simulink model "HW2_FSR_ES3_Almost_NonLinear"  (R2023b)
settings: Solver=ode23  StartTime=0.0  StopTime=T  FixedStep=0.001  RelTol=1e-5
values from neighbouring files (symbols this model uses):
  c = 36/r^0.3    (= 36)    [HW2_FSR_ES3.m]
  k_2_a = 3*c^2/r    (= 3888)    [HW2_FSR_ES3.m]
  r = 1    [HW2_FSR_ES3.m]
libraries: robotmobilelib x1
settings Model: Creator=emman  LastModifiedBy=emman

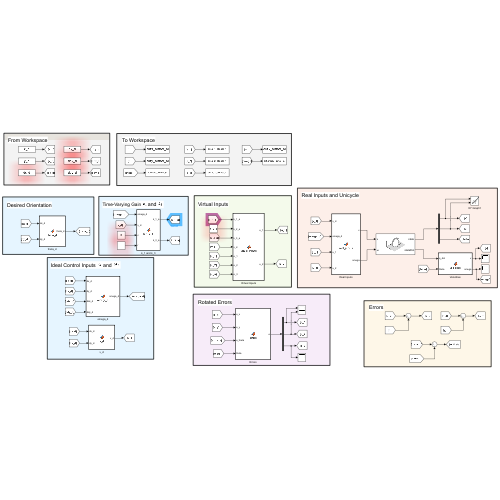
[thumbnail: Simulink's stored preview of the top-level diagram]
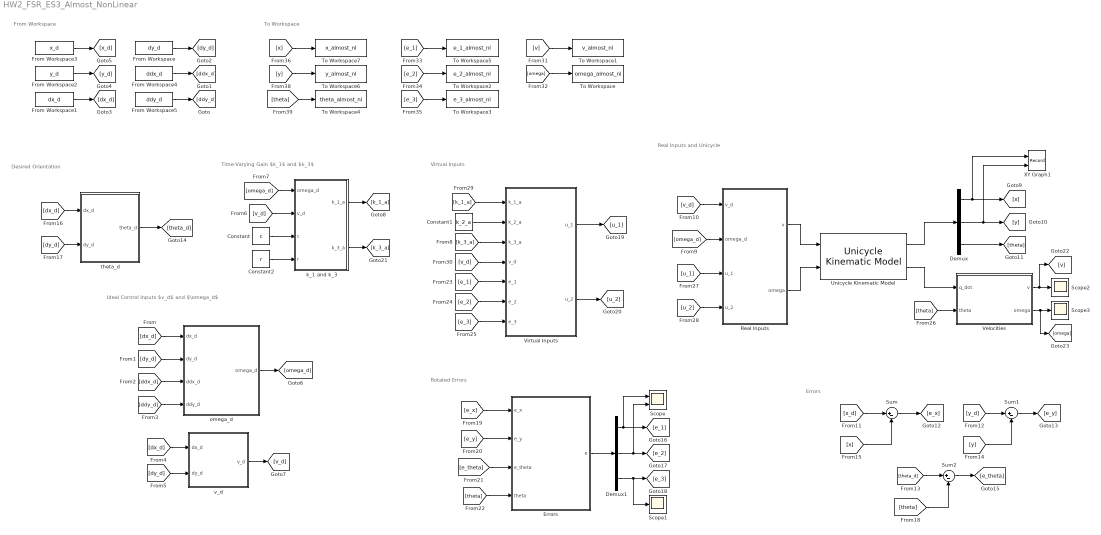
== system HW2_FSR_ES3_Almost_NonLinear ==
  note: To Workspace
  note: From Workspace
  note: Desired Orientation
  note: Rotated Errors
  note: Ideal Control Inputs $v_d$ and $\omega_d$
  note: Time-Varying Gain $k_1$ and $k_3$
  note: Virtual Inputs
  note: Real Inputs and Unicycle
  note: Errors
  Constant : Constant  Value=c
  Constant1 : Constant  Value=k_2_a
  Constant2 : Constant  Value=r
  Demux : Demux  Outputs=3
  Demux1 : Demux  Outputs=3
  Errors : MATLAB Function  TreatAsAtomicUnit=on
  From Workspace : FromWorkspace  VariableName=dy_d
  From Workspace1 : FromWorkspace  VariableName=dx_d
  From Workspace2 : FromWorkspace  VariableName=y_d
  From Workspace3 : FromWorkspace  VariableName=x_d
  From Workspace4 : FromWorkspace  VariableName=ddx_d
  From Workspace5 : FromWorkspace  VariableName=ddy_d
  Real Inputs : MATLAB Function  TreatAsAtomicUnit=on
  Scope : Scope  NumInputPorts=2
  Scope1 : Scope
  Scope2 : Scope
  Scope3 : Scope
  Sum : Sum  Inputs=|+-
  Sum1 : Sum  Inputs=|+-
  Sum2 : Sum  Inputs=|+-
  To Workspace : ToWorkspace  VariableName=omega_almost_nl  SaveFormat=Timeseries  SampleTime=-1
  To Workspace1 : ToWorkspace  VariableName=v_almost_nl  SaveFormat=Timeseries  SampleTime=-1
  To Workspace2 : ToWorkspace  VariableName=e_2_almost_nl  SaveFormat=Timeseries  SampleTime=-1
  To Workspace3 : ToWorkspace  VariableName=e_3_almost_nl  SaveFormat=Timeseries  SampleTime=-1
  To Workspace4 : ToWorkspace  VariableName=theta_almost_nl  SaveFormat=Timeseries  SampleTime=-1
  To Workspace5 : ToWorkspace  VariableName=e_1_almost_nl  SaveFormat=Timeseries  SampleTime=-1
  To Workspace6 : ToWorkspace  VariableName=y_almost_nl  SaveFormat=Timeseries  SampleTime=-1
  To Workspace7 : ToWorkspace  VariableName=x_almost_nl  SaveFormat=Timeseries  SampleTime=-1
  Unicycle Kinematic Model : robotmobilelib/Unicycle Kinematic Model  VehicleInputs=Vehicle Speed & Heading Angular Velocity  WheelRadius=0.1  WheelSpeedRange=[-Inf Inf]  InitialState=q_i  SimulateUsing=Interpreted execution
  Velocities : MATLAB Function  TreatAsAtomicUnit=on
  Virtual Inputs : MATLAB Function  TreatAsAtomicUnit=on
  XY Graph1 : Record  FileSettingsInternal="{\"entries\":[{\"content\":{\"excelSettings\":{\"content\":{},\"type\":\"Streamout.ExcelSettings\"}},\"type\":\"Streamout.FileSettingStorage\",\"uuid\":\"\"}],\"packageUris\":[\"http:\\/\\/schema.mathworks.com\\/mf0\\/streamout_blocks\\/R2020a\"],\"version\":\"1.0\"}"  Layout=[1 1]  SignalsInternal="{\"entries\":[{\"content\":{\"signals\":[{\"content\":{\"blockPath\":[],\"dimensions\":[1],\"domain\":\"\",\"lineColor\":\"#77ac30\",\"plots\":[1],\"port\":1,\"sid\":[\"\"],\"signalID\":6338,\"signalName\":\"Demux:1\"},\"type\":\"RecordBlkView.Signal\",\"uuid\":\"\"},{\"content\":{\"blockPath\":[],\"dimensions\":[1],\"domain\":\"\",\"lineColor\":\"#4dbeee\",\"plots\":[1],\"port\":2,\"sid\":[\"\"],\"signalID\":6342,\"signalName\":\"Demux:2\"},\"type\":\"RecordBlkView.Signal\",\"uuid\":\"\"}]},\"type\":\"RecordBlkView.InputSignals\",\"uuid\":\"\"}],\"packageUris\":[\"http:\\/\\/schema.mathworks.com\\/mf0\\/streamout_blocks\\/R2020a\"],\"version\":\"1.0\"}"  VisualizationBindings="{\"xyplotplugin\":{\"info\":[{\"series\":[{\"bindingParametersList\":[{\"parameter\":\"X-Axis\",\"signalID\":6338,\"signalName\":\"Demux:1\"},{\"parameter\":\"Y-Axis\",\"signalID\":6342,\"signalName\":\"Demux:2\"}],\"seriesID\":27378}],\"subplotID\":1}]}}"  CompatibilityTag=XY  st=-1
  k_1 and k_3 : MATLAB Function  TreatAsAtomicUnit=on
  omega_d : MATLAB Function  TreatAsAtomicUnit=on
  theta_d : MATLAB Function  TreatAsAtomicUnit=on
  v_d : MATLAB Function  TreatAsAtomicUnit=on
  wires:
  Unicycle Kinematic Model/1 -> Demux/1
  Sum1/1 -> [e_y]
  From Workspace1/1 -> [dx_d]
  [theta] -> Sum2/2
  [e_1] -> Virtual Inputs/5(e_1)
  Unicycle Kinematic Model/2 -> Velocities/1(q_dot)
  [ddx_d] -> omega_d/3(ddx_d)
  [e_3] -> Virtual Inputs/7(e_3)
  [dy_d] -> omega_d/2(dy_d)
  Velocities/1(v) -> [v], Scope2/1
  Demux/2 -> [y], XY Graph1/2
  Velocities/2(omega) -> [omega], Scope3/1
  Virtual Inputs/1(u_1) -> [u_1]
  [u_2] -> Real Inputs/4(u_2)
  Virtual Inputs/2(u_2) -> [u_2]
  k_1 and k_3/1(k_1_a) -> [k_1_a]
  Real Inputs/1(v) -> Unicycle Kinematic Model/1
  Demux/1 -> [x], XY Graph1/1
  [k_3_a] -> Virtual Inputs/3(k_3_a)
  Constant1/1 -> Virtual Inputs/2(k_2_a)
  Demux1/3 -> Scope1/1, [e_3]
  [dx_d] -> v_d/1(dx_d)
  Real Inputs/2(omega) -> Unicycle Kinematic Model/2
  [omega_d] -> Real Inputs/2(omega_d)
  [v_d] -> k_1 and k_3/2(v_d)
  [theta] -> Velocities/2(theta)
  v_d/1(v_d) -> [v_d]
  omega_d/1(omega_d) -> [omega_d]
  [omega_d] -> k_1 and k_3/1(omega_d)
  [dx_d] -> omega_d/1(dx_d)
  [u_1] -> Real Inputs/3(u_1)
  [dy_d] -> v_d/2(dy_d)
  Demux1/1 -> Scope/1, [e_1]
  [ddy_d] -> omega_d/4(ddy_d)
  Constant/1 -> k_1 and k_3/3(c)
  From Workspace2/1 -> [y_d]
  From Workspace4/1 -> [ddx_d]
  From Workspace5/1 -> [ddy_d]
  Demux1/2 -> Scope/2, [e_2]
  [e_2] -> Virtual Inputs/6(e_2)
  [theta_d] -> Sum2/1
  [theta] -> Errors/4(theta)
  [e_x] -> Errors/1(e_x)
  [x] -> Sum/2
  theta_d/1(theta_d) -> [theta_d]
  [e_y] -> Errors/2(e_y)
  From Workspace/1 -> [dy_d]
  Sum/1 -> [e_x]
  [y_d] -> Sum1/1
  [dy_d] -> theta_d/2(dy_d)
  Sum2/1 -> [e_theta]
  [v_d] -> Real Inputs/1(v_d)
  Demux/3 -> [theta]
  Errors/1(e) -> Demux1/1
  [e_theta] -> Errors/3(e_theta)
  From Workspace3/1 -> [x_d]
  [k_1_a] -> Virtual Inputs/1(k_1_a)
  [y] -> Sum1/2
  [x_d] -> Sum/1
  [dx_d] -> theta_d/1(dx_d)
  k_1 and k_3/2(k_3_a) -> [k_3_a]
  [v_d] -> Virtual Inputs/4(v_d)
  Constant2/1 -> k_1 and k_3/4(r)
  [x] -> To Workspace7/1
  [y] -> To Workspace6/1
  [theta] -> To Workspace4/1
  [e_1] -> To Workspace5/1
  [e_2] -> To Workspace2/1
  [e_3] -> To Workspace3/1
  [v] -> To Workspace1/1
  [omega] -> To Workspace/1

== matlab function HW2_FSR_ES3_Almost_NonLinear/omega_d ==
  data: dx_d input; omega_d output; dy_d input; ddx_d input; ddy_d input
function omega_d  = omega_d(dx_d, dy_d, ddx_d, ddy_d)

omega_d = (ddy_d.*dx_d - ddx_d.*dy_d)./(dx_d.^2 + dy_d.^2);

== matlab function HW2_FSR_ES3_Almost_NonLinear/Virtual Inputs ==
  data: k_1_a input; u_1 output; k_2_a input; k_3_a input; v_d input; e_1 input; e_2 input; e_3 input; u_2 output
function [u_1, u_2] = virtual_inputs(k_1_a, k_2_a, k_3_a, v_d, e_1, e_2, e_3)

u_1 = -k_1_a*e_1;
u_2 = -k_2_a*v_d*(sin(e_3)/e_3)*e_2 - k_3_a*e_3;

== matlab function HW2_FSR_ES3_Almost_NonLinear/k_1 and k_3 ==
  data: omega_d input; k_1_a output; v_d input; c input; k_3_a output; r input
function [k_1_a, k_3_a] = k_1_3_a(omega_d, v_d, c, r)

%k_1_a = (c^2 - omega_d)/v_d;
%k_3_a = k_1_a;

k_1_a = r^2*c^2*sqrt(v_d^2 + omega_d^2)/v_d^2;
k_3_a = k_1_a;

== matlab function HW2_FSR_ES3_Almost_NonLinear/v_d ==
  data: dx_d input; v_d output; dy_d input
function v_d = v_d(dx_d, dy_d)

v_d = sqrt(dx_d^2 + dy_d^2);

== matlab function HW2_FSR_ES3_Almost_NonLinear/Real Inputs ==
  data: v_d input; v output; omega_d input; u_1 input; u_2 input; omega output
function [v, omega] = real_inputs(v_d, omega_d, u_1, u_2)

v = v_d - u_1;
omega = omega_d - u_2;

== matlab function HW2_FSR_ES3_Almost_NonLinear/theta_d ==
  data: dx_d input; theta_d output; dy_d input
function theta_d = theta_d(dx_d, dy_d)

theta_d = atan2(dy_d, dx_d);

== matlab function HW2_FSR_ES3_Almost_NonLinear/Errors ==
  data: e_x input; e output; e_y input; e_theta input; theta input
function e = errors(e_x, e_y, e_theta, theta)

R = [cos(theta) sin(theta) 0; 
    -sin(theta) cos(theta) 0;
    0 0 1];

e = R*[e_x; e_y; e_theta];

== matlab function HW2_FSR_ES3_Almost_NonLinear/Velocities ==
  data: q_dot input; v output; theta input; omega output
function [v, omega] = velocities(q_dot, theta)

v = q_dot(1)/cos(theta);
omega = q_dot(3);
